simulink model "simulate_robot_and_motors"  (R2015a)
settings: Solver=ode23  StartTime=0.0  StopTime=10  FixedStep=0.005  RelTol=1e-3
values from neighbouring files (symbols this model uses):
  robot = load_robot('example','2dofplanar')    [runge_kutta_exercises.m]
undefined symbols (not defined in the file or in its folder): call_direct_dynamics_2dofplanar, call_third_order_planner
settings Model: Creator=arturo  LastModifiedBy=arturogilaparicio
settings DataIOCC: LimitDataPoints=off  SignalLoggingSaveFormat=ModelDataLogs
settings OptimizationCC: ExpressionDepthLimit=2147483647
settings DebuggingCC: UnderspecifiedInitializationDetection=Classic  MergeDetectMultiDrivingBlocksExec=none  SolverPrmCheckMsg=warning  FcnCallInpInsideContextMsg=EnableAllAsWarning  StateNameClashWarn=warning
settings SFSimCC: SimParseCustomCode=off
settings GRTTargetCC: CombineOutputUpdateFcns=off  GRTInterface=on

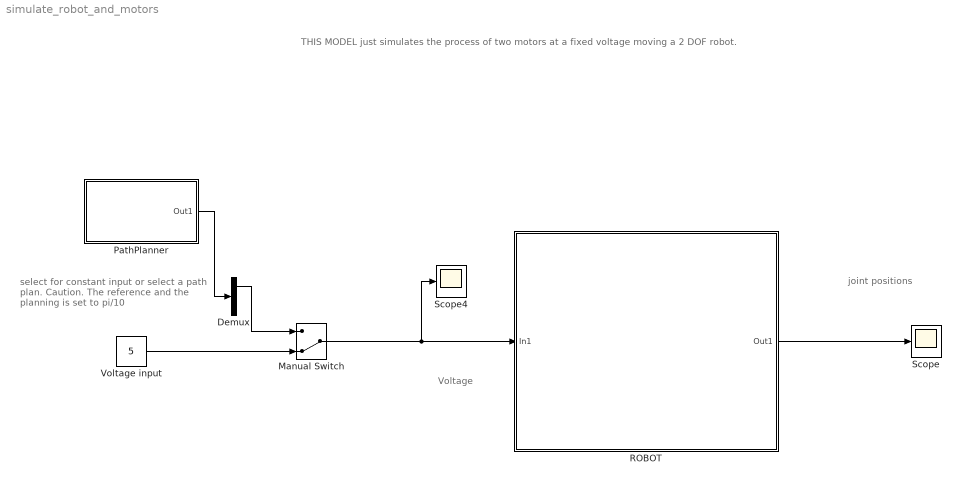
== system simulate_robot_and_motors ==
  note: THIS MODEL just simulates the process of two motors at a fixed voltage moving a 2 DOF robot.
  note: select for constant input or select
      | a path plan. Caution. The reference and
      | the planning is set to pi/10
  note: Voltage
  note: joint positions
  Demux : Demux  Outputs=3
  Manual Switch : ManualSwitch  CurrentSetting=0
  PathPlanner : Subsystem
      mask Display: port_label('output', 1, 'q, qd, qdd')
  ROBOT : Subsystem
      mask Display: image(imread('images/robot2dof.png'))
  Scope : Scope
      settings: TimeRange=2  YMin=0.1125  YMax=0.1575
  Scope4 : Scope
      settings: YMin=-2.5  YMax=50  SaveName=ScopeData4
  "Voltage input " : Constant  Value=5
  wires:
  Manual Switch/1 -> ROBOT/1(In1), Scope4/1
  ROBOT/1(Out1) -> Scope/1
  PathPlanner/1(Out1) -> Demux/1
  "Voltage input "/1 -> Manual Switch/2
  Demux/1 -> Manual Switch/1

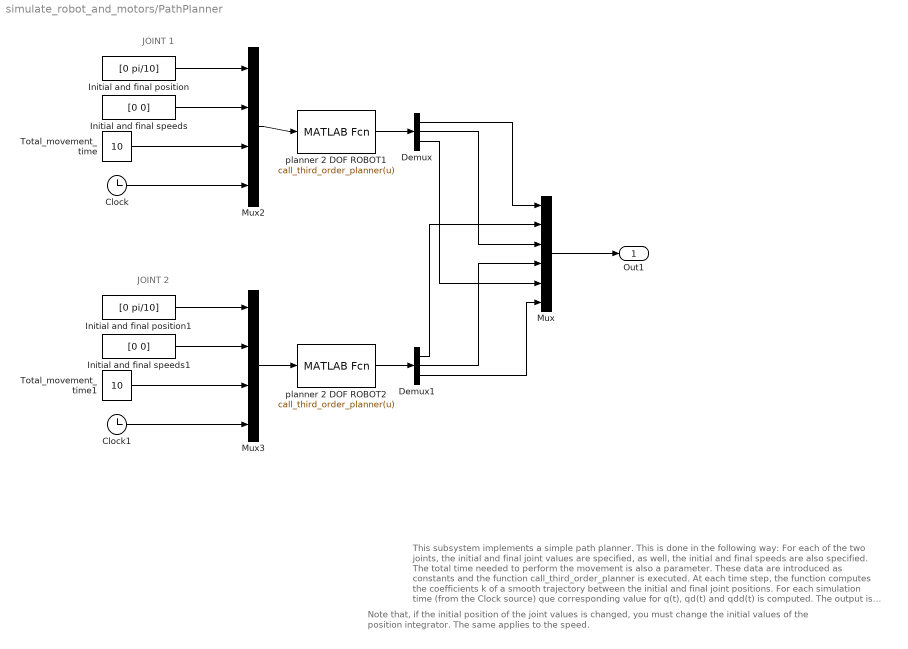
== system simulate_robot_and_motors/PathPlanner ==
  note: JOINT 1
  note: JOINT 2
  note: This subsystem implements a simple path planner. This is done in the following way: For each of the two joints,
      | the initial and final joint values are specified, as well, the initial and final speeds are also specified. The total time needed to perform the movement is also
      | a parameter. These data are introduced as constants and the function call_third_order_planner is executed. At each time step, the function computes the coefficients
      | k of a smooth trajectory between the initial and final joint positions. For each simulation time (from the Clock source) que corresponding value for q(t), qd(t) and qdd(t) is computed.
      | The output is formed by 6 variables (2 values of position, 2 of joint speed and 2 of acceleration)
  note: Note that, if the initial position of the joint values is changed, you must change the initial values of the position integrator. The same applies to the speed.
  Clock : Clock
  Clock1 : Clock
  Demux : Demux  Outputs=3
  Demux1 : Demux  Outputs=3
  Initial and final position : Constant  Value=[0 pi/10]
  Initial and final position1 : Constant  Value=[0 pi/10]
  Initial and final speeds : Constant  Value=[0 0]
  Initial and final speeds1 : Constant  Value=[0 0]
  Mux : Mux  Inputs=6
  Mux2 : Mux
  Mux3 : Mux
  Total_movement_time : Constant  Value=10
  Total_movement_time1 : Constant  Value=10
  planner 2 DOF ROBOT1 : MATLABFcn  MATLABFcn=call_third_order_planner(u)  OutputDimensions=3
  planner 2 DOF ROBOT2 : MATLABFcn  MATLABFcn=call_third_order_planner(u)  OutputDimensions=3
  Out1 : Outport
  wires:
  Initial and final position/1 -> Mux2/1
  Initial and final speeds/1 -> Mux2/2
  Total_movement_time/1 -> Mux2/3
  Clock/1 -> Mux2/4
  Mux2/1 -> planner 2 DOF ROBOT1/1
  Initial and final position1/1 -> Mux3/1
  Initial and final speeds1/1 -> Mux3/2
  Total_movement_time1/1 -> Mux3/3
  Clock1/1 -> Mux3/4
  Mux3/1 -> planner 2 DOF ROBOT2/1
  planner 2 DOF ROBOT1/1 -> Demux/1
  planner 2 DOF ROBOT2/1 -> Demux1/1
  Demux/1 -> Mux/1
  Demux1/1 -> Mux/2
  Demux/2 -> Mux/3
  Demux1/2 -> Mux/4
  Demux/3 -> Mux/5
  Demux1/3 -> Mux/6
  Mux/1 -> Out1/1

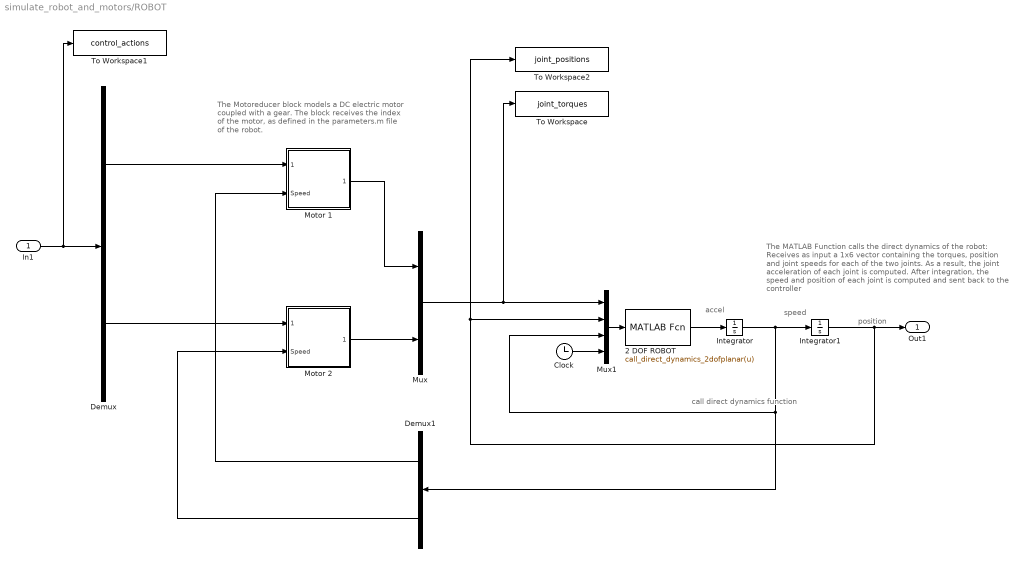
== system simulate_robot_and_motors/ROBOT ==
  note: accel
  note: speed
  note: position
  note: The MATLAB Function calls the direct dynamics of the robot:
      | Receives as input a 1x6 vector containing the
      | torques, position and joint
      | speeds for each of the two joints. As a result, the joint
      | acceleration of each joint is computed.
      | After integration, the speed and position of each joint
      | is computed and sent back to the controller
  note: call direct dynamics
      |  function
  note: The Motoreducer block models a DC
      | electric motor coupled with a gear.
      | The block receives the index of the motor,
      | as defined in the parameters.m file of the robot.
  In1 : Inport
  2 DOF ROBOT : MATLABFcn  MATLABFcn=call_direct_dynamics_2dofplanar(u)  OutputDimensions=2
  Clock : Clock
  Demux : Demux  Outputs=2
  Demux1 : Demux  Outputs=2
  Integrator : Integrator  InitialCondition=[0 0 ]
  Integrator1 : Integrator  InitialCondition=[0 0]
  Motor 1 : Subsystem
  Motor 2 : Subsystem
  Mux : Mux  Inputs=2
  Mux1 : Mux
  To Workspace : ToWorkspace  VariableName=joint_torques  SampleTime=-1
  To Workspace1 : ToWorkspace  VariableName=control_actions  SampleTime=-1
  To Workspace2 : ToWorkspace  VariableName=joint_positions  SampleTime=-1
  Out1 : Outport
  wires:
  Demux/1 -> Motor 1/1(Input (Volts))
  Demux/2 -> Motor 2/1(Input (Volts))
  Mux1/1 -> 2 DOF ROBOT/1
  2 DOF ROBOT/1 -> Integrator/1
  Integrator/1 -> Integrator1/1, Demux1/1, Mux1/3
  Motor 1/1(Output Torque) -> Mux/1
  Demux1/1 -> Motor 1/2(Speed)
  Motor 2/1(Output Torque) -> Mux/2
  Demux1/2 -> Motor 2/2(Speed)
  In1/1 -> To Workspace1/1, Demux/1
  Integrator1/1 -> Out1/1, Mux1/2, To Workspace2/1
  Mux/1 -> Mux1/1, To Workspace/1
  Clock/1 -> Mux1/4

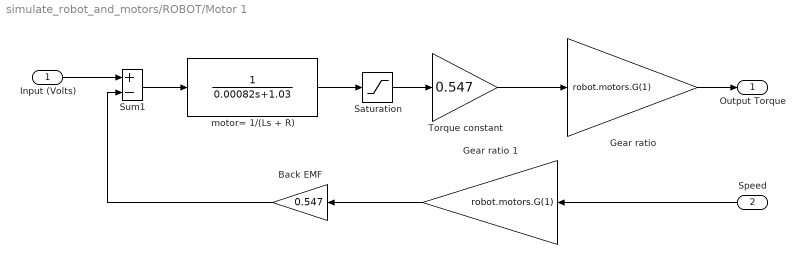
== system simulate_robot_and_motors/ROBOT/Motor 1 ==
  Input (Volts) : Inport
  Speed : Inport  Port=2
  Back EMF : Gain  Gain=0.547  SaturateOnIntegerOverflow=on  OutDataTypeStr=Inherit: Same as input  ParamDataTypeStr=Inherit: Same as input
  Gear ratio : Gain  Gain=robot.motors.G(1)  SaturateOnIntegerOverflow=on  OutDataTypeStr=Inherit: Same as input  ParamDataTypeStr=Inherit: Same as input
  Gear ratio 1 : Gain  Gain=robot.motors.G(1)  SaturateOnIntegerOverflow=on  OutDataTypeStr=Inherit: Same as input  ParamDataTypeStr=Inherit: Same as input
  Saturation : Saturate  UpperLimit=30  LowerLimit=-30  ZeroCross=off
  Sum1 : Sum  Inputs=+-  SaturateOnIntegerOverflow=on  InputSameDT=on  OutDataTypeStr=Inherit: Same as first input
  Torque constant : Gain  Gain=0.547  SaturateOnIntegerOverflow=on  OutDataTypeStr=Inherit: Same as input  ParamDataTypeStr=Inherit: Same as input
  motor= 1/(Ls + R) : TransferFcn  Denominator=[0.00082 1.03]
  Output Torque : Outport  InitialOutput=0
  wires:
  Gear ratio 1/1 -> Back EMF/1
  Speed/1 -> Gear ratio 1/1
  Input (Volts)/1 -> Sum1/1
  Back EMF/1 -> Sum1/2
  Sum1/1 -> motor= 1/(Ls + R)/1
  Gear ratio/1 -> Output Torque/1
  Torque constant/1 -> Gear ratio/1
  motor= 1/(Ls + R)/1 -> Saturation/1
  Saturation/1 -> Torque constant/1

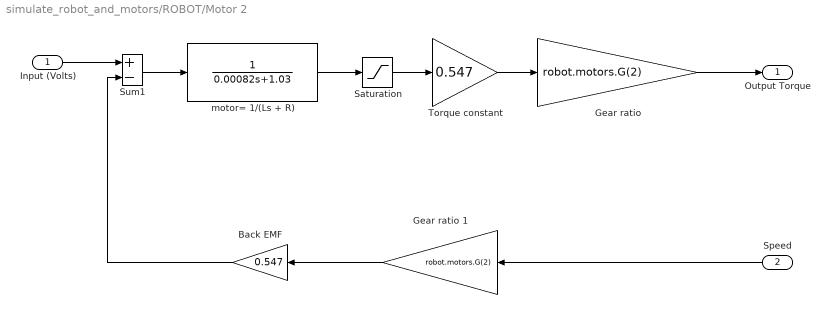
== system simulate_robot_and_motors/ROBOT/Motor 2 ==
  Input (Volts) : Inport
  Speed : Inport  Port=2
  Back EMF : Gain  Gain=0.547  SaturateOnIntegerOverflow=on  OutDataTypeStr=Inherit: Same as input  ParamDataTypeStr=Inherit: Same as input
  Gear ratio : Gain  Gain=robot.motors.G(2)  SaturateOnIntegerOverflow=on  OutDataTypeStr=Inherit: Same as input  ParamDataTypeStr=Inherit: Same as input
  Gear ratio 1 : Gain  Gain=robot.motors.G(2)  SaturateOnIntegerOverflow=on  OutDataTypeStr=Inherit: Same as input  ParamDataTypeStr=Inherit: Same as input
  Saturation : Saturate  UpperLimit=30  LowerLimit=-30  ZeroCross=off
  Sum1 : Sum  Inputs=+-  SaturateOnIntegerOverflow=on  InputSameDT=on  OutDataTypeStr=Inherit: Same as first input
  Torque constant : Gain  Gain=0.547  SaturateOnIntegerOverflow=on  OutDataTypeStr=Inherit: Same as input  ParamDataTypeStr=Inherit: Same as input
  motor= 1/(Ls + R) : TransferFcn  Denominator=[0.00082 1.03]
  Output Torque : Outport  InitialOutput=0
  wires:
  Saturation/1 -> Torque constant/1
  motor= 1/(Ls + R)/1 -> Saturation/1
  Torque constant/1 -> Gear ratio/1
  Gear ratio/1 -> Output Torque/1
  Sum1/1 -> motor= 1/(Ls + R)/1
  Back EMF/1 -> Sum1/2
  Input (Volts)/1 -> Sum1/1
  Speed/1 -> Gear ratio 1/1
  Gear ratio 1/1 -> Back EMF/1
